simulink model "Float_point"  (R2022b)
settings: Solver=VariableStepAuto  StartTime=0.0  StopTime=10.0  RelTol=1e-3
settings Model: Creator=Sonikot  LastModifiedBy=Sonikot

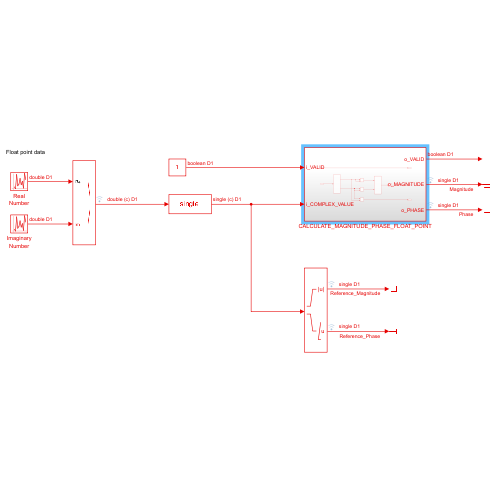
[thumbnail: Simulink's stored preview of the top-level diagram]
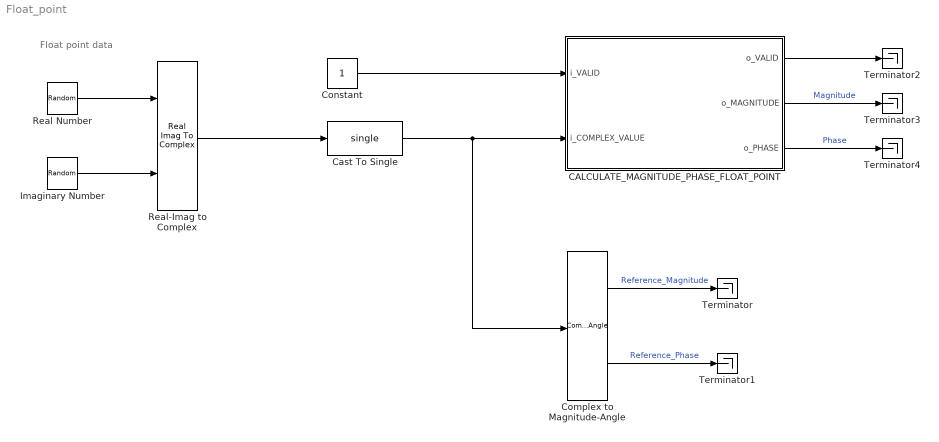
== system Float_point ==
  note: Float point data
  CALCULATE_MAGNITUDE_PHASE_FLOAT_POINT : Subsystem
  Cast To Single : DataTypeConversion  OutDataTypeStr=single  SaturateOnIntegerOverflow=off  RndMeth=Floor
  Complex to Magnitude-Angle : ComplexToMagnitudeAngle
  Constant : Constant  OutDataTypeStr=boolean  SampleTime=1
  Imaginary Number : UniformRandomNumber  Minimum=0  Maximum=255.99999994039535522461  Seed=9  SampleTime=1
  Real Number : UniformRandomNumber  Minimum=0  Maximum=255.99999994039535522461  Seed=8  SampleTime=1
  Real-Imag to Complex : RealImagToComplex
  Terminator{,1..4} (5 alike) : Terminator
  wires:
  CALCULATE_MAGNITUDE_PHASE_FLOAT_POINT/3(o_PHASE) -> Terminator4/1  "Phase"
  Constant/1 -> CALCULATE_MAGNITUDE_PHASE_FLOAT_POINT/1(i_VALID)
  CALCULATE_MAGNITUDE_PHASE_FLOAT_POINT/1(o_VALID) -> Terminator2/1
  CALCULATE_MAGNITUDE_PHASE_FLOAT_POINT/2(o_MAGNITUDE) -> Terminator3/1  "Magnitude"
  Cast To Single/1 -> Complex to Magnitude-Angle/1, CALCULATE_MAGNITUDE_PHASE_FLOAT_POINT/2(i_COMPLEX_VALUE)
  Imaginary Number/1 -> Real-Imag to Complex/2
  Real-Imag to Complex/1 -> Cast To Single/1
  Complex to Magnitude-Angle/1 -> Terminator/1  "Reference_Magnitude"
  Complex to Magnitude-Angle/2 -> Terminator1/1  "Reference_Phase"
  Real Number/1 -> Real-Imag to Complex/1

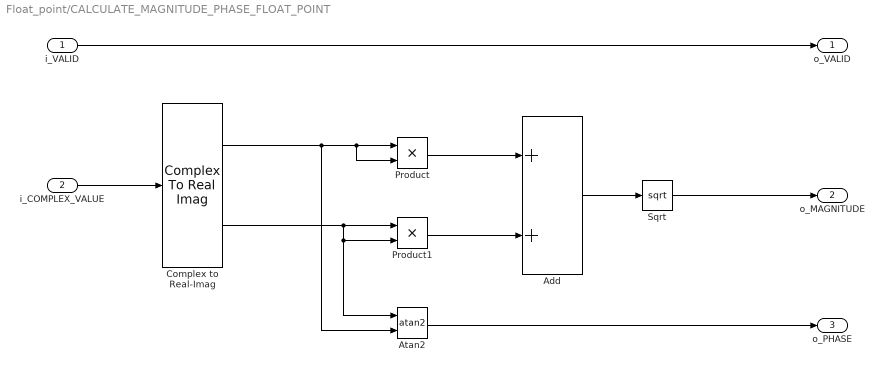
== system Float_point/CALCULATE_MAGNITUDE_PHASE_FLOAT_POINT ==
  i_VALID : Inport
  i_COMPLEX_VALUE : Inport  Port=2
  Add : Sum
  Atan2 : Trigonometry  Operator=atan2  NumberOfIterations=20
  Complex to Real-Imag : ComplexToRealImag
  Product : Product
  Product1 : Product
  Sqrt : Sqrt
  o_VALID : Outport
  o_MAGNITUDE : Outport  Port=2
  o_PHASE : Outport  Port=3
  wires:
  Sqrt/1 -> o_MAGNITUDE/1
  i_VALID/1 -> o_VALID/1
  Add/1 -> Sqrt/1
  i_COMPLEX_VALUE/1 -> Complex to Real-Imag/1
  Product1/1 -> Add/2
  Product/1 -> Add/1
  Complex to Real-Imag/1 -> Atan2/2, Product/2, Product/1
  Complex to Real-Imag/2 -> Product1/1, Atan2/1, Product1/2
  Atan2/1 -> o_PHASE/1
